simulink model "KD_cl_harness_tomasso"  (R2014b)
settings: Solver=ode45  StartTime=0  StopTime=50  FixedStep=0.01  MaxStep=0.005  RelTol=1e-4  AbsTol=1e-4
InitFcn:
  | load KD_const_coeffs_0624
  | load pexhat_stuff
  | load expcon
  | load thr_ff_map
values from neighbouring files (symbols this model uses):
  c_0 = 0    [expcon.mat]
  c_1 = 1    [expcon.mat]
  c_100 = 100    [expcon.mat]
  c_1000 = 1000    [expcon.mat]
  c_10000 = 10000    [expcon.mat]
  c_1000inv = 0.0010000000475    [expcon.mat]    (also in pexhat_stuff.mat)
  c_100inv = 0.00999999977648    [expcon.mat]
  c_1_int = 1    [expcon.mat]
  c_1d2p4 = 0.416666656733    [expcon.mat]
  c_1p7 = 1.70000004768    [expcon.mat]
  c_4400inv = 0.000227272728807    [pexhat_stuff.mat]
  c_5500inv = 0.000181818177225    [expcon.mat]
  c_80 = 80    [expcon.mat]
  c_90 = 90    [expcon.mat]
  c_cal_phi = 7.6395999713e-06    [expcon.mat]
  c_compmap = [28125.0058594 29577.4082031 31350.1035156 33776.21875 37051.9296875 41026.2695312 45453.9960938 50160.3515625 55029.671875 59986.109375 64980.4296875 69980.4375 ... (320 elements, 20x16)]    [expcon.mat]
  c_ctok = 273.149993896    [expcon.mat]
  c_fflow_max = inf    [expcon.mat]
  c_fflow_min = 0    [expcon.mat]
  c_filt = 0.949999988079    [expcon.mat]
  c_flowdiv = 9.99999974738e-05    [expcon.mat]
  c_flowmin = 0    [expcon.mat]
  c_flowmult = 10000    [expcon.mat]
  c_inf = inf    [expcon.mat]
  c_km1d2k = 0.142857149243    [expcon.mat]
  c_mm3tokgpers = 2.77333338516e-08    [expcon.mat]
  c_n1 = -1    [expcon.mat]
  c_p00001 = 9.99999974738e-06    [expcon.mat]
  c_p01 = 0.00999999977648    [pexhat_stuff.mat]
  c_p016 = 0.01600000076    [expcon.mat]
  c_p1429 = 0.142900004983    [expcon.mat]
  c_p1e9 = 9.99999971718e-10    [expcon.mat]
  c_p4167 = 0.416700005531    [expcon.mat]    (also in pexhat_stuff.mat = 0.416666656733)
  c_p4d1p4 = 0.285714298487    [expcon.mat]
  c_p5401 = 0.540099978447    [expcon.mat]
  c_p9 = 0.899999976158    [expcon.mat]
  c_pincomp = 97.4216003418    [expcon.mat]
  c_ra = 287.002807617    [expcon.mat]
  c_rair = 287.09979248    [expcon.mat]
  c_Rby1000 = 0.000287000002572    [expcon.mat]
  c_roacorr = 8.05689978733e-06    [expcon.mat]
  c_rpmtoradpers = 0.104719758034    [expcon.mat]
  c_svrthrottle1 = [0.924875080585 0.575991511345 0.0858279466629 0.820202827454 0.445821881294 0.509882986546 0.0428557097912 0.753634572029 0]    [expcon.mat]
  c_svrthrottle2 = [0.145454958081 0.14545533061 0.363636374474 0.509091556072 0.509090721607 0.509091317654 0.545454084873 0.618182241917 0.145454272628]    [expcon.mat]
  c_svrthrottlearg = 0.10000000149    [expcon.mat]
  c_svrthrottlebeta = [2282.12670898 -3239.46044922 -142.784469604 -2660.34570312 1434.34350586 4150.43994141 -1580.68164062 -1039.89575195 791.34588623]    [expcon.mat]
  c_ta_max = inf    [expcon.mat]
  c_ta_min = 270    [expcon.mat]
  c_V = 0.0077999997884    [expcon.mat]
  c_vnliftmax = 90    [expcon.mat]
  c_vnliftmin = 40    [expcon.mat]
  Coefs =     [KD_const_coeffs_0624.mat]    (also in pexhat_stuff.mat)
  const =     [KD_const_coeffs_0624.mat]    (also in pexhat_stuff.mat)
  const_exhat =     [pexhat_stuff.mat]
  eegr_map =     [expcon.mat]
  egrr_delay_init = 0    [expcon.mat]
  epim_map =     [expcon.mat]
  eplufin_ff_map =     [expcon.mat]
  expcon =     [expcon.mat]
  invta = [5 5 5 5 2.5 0 0 0 0 0 0 0 ... (240 elements, 16x15)]    [expcon.mat]
  invtacols = [1000 1200 1400 1600 1800 2000 2200 2400 2600 2800 3000 3200 ... (16 elements, 1x16)]    [expcon.mat]
  IV =     [KD_const_coeffs_0624.mat]    (also in pexhat_stuff.mat)
  Lobs_init = [0 0 0]    [expcon.mat]
  map_delay_init = 120    [expcon.mat]
  maxA_t = [51.4567184448 53.8593139648 56.3063011169 58.7576789856 61.1701469421 63.4982337952 65.6955718994 67.7161483765 69.5156555176 71.0527648926 72.2902603149 73.1961746216 ... (16 elements, 1x16)]    [expcon.mat]
  obsA = [0.985195398331  0  0; -0.188821405172  1  0; 0.000342977960827  0  1]    [expcon.mat]
  sample_time = 0.016    [expcon.mat]    (also in pexhat_stuff.mat)
  SVR_EGR =     [KD_const_coeffs_0624.mat]    (also in pexhat_stuff.mat)
  SVR_EGR_exhat =     [pexhat_stuff.mat]
  SVR_throttle =     [KD_const_coeffs_0624.mat]    (also in pexhat_stuff.mat)
  uz_init = [0 0]    [expcon.mat]
undefined symbols (not defined in the file or in its folder): k1_table, k2_table, maxL, minL, Newton, Raphson
libraries: simulink x5
(part 2 of 6)

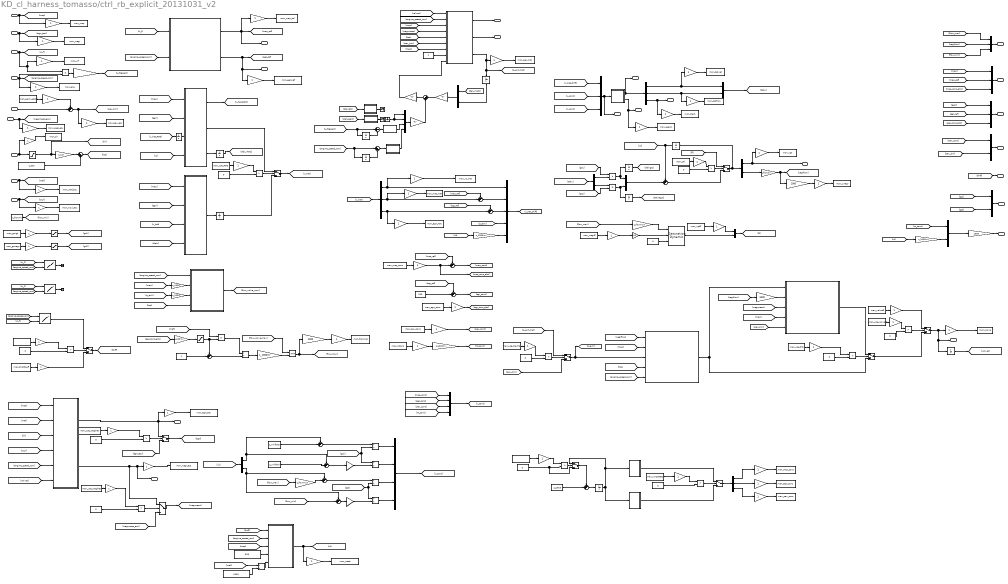
== system KD_cl_harness_tomasso/ctrl_rb_explicit_20131031_v2 ==
  map_kPa : Inport  OutDataTypeStr=single  PortDimensions=1  SampleTime=sample_time
  egrr_ecu : Inport  Port=2  OutDataTypeStr=single  PortDimensions=1  SampleTime=sample_time
  u_fuel_mm3pst : Inport  Port=3  OutDataTypeStr=single  PortDimensions=1  SampleTime=sample_time
  ene_rpm : Inport  Port=4  OutDataTypeStr=single  PortDimensions=1  SampleTime=sample_time
  pexh_kpa : Inport  Port=5  OutDataTypeStr=single  PortDimensions=1  SampleTime=sample_time
  t_in_C : Inport  Port=6  OutDataTypeStr=single  PortDimensions=1  SampleTime=sample_time
  wegrmeas_gps : Inport  Port=7  OutDataTypeStr=single  PortDimensions=1  SampleTime=sample_time
  maf_gps : Inport  Port=8  OutDataTypeStr=single  PortDimensions=1  SampleTime=sample_time
  wcyl : Inport  Port=9  OutDataTypeStr=single  PortDimensions=1  SampleTime=sample_time
  Data Store Read : DataStoreRead  DataStoreName=man_gsvgt  SampleTime=sample_time
  Data Store Read1 : DataStoreRead  DataStoreName=man_gswegr  SampleTime=sample_time
  Data Store Read10 : DataStoreRead  DataStoreName=man_use_valveff  SampleTime=sample_time
  Data Store Read11 : DataStoreRead  DataStoreName=man_valveff  SampleTime=sample_time
  Data Store Read12 : DataStoreRead  DataStoreName=man_use_throttleffmap  SampleTime=sample_time
  Data Store Read13 : DataStoreRead  DataStoreName=man_use_PexHat  SampleTime=sample_time
  Data Store Read14 : DataStoreRead  DataStoreName=man_pexh_adder  SampleTime=sample_time
  Data Store Read15 : DataStoreRead  DataStoreName=man_use_PID  SampleTime=sample_time
  Data Store Read16 : DataStoreRead  DataStoreName=man_use_ROO  SampleTime=sample_time
  Data Store Read17 : DataStoreRead  DataStoreName=man_pex_cons  SampleTime=sample_time
  Data Store Read18 : DataStoreRead  DataStoreName=man_ntcons  SampleTime=sample_time
  Data Store Read19 : DataStoreRead  DataStoreName=man_run2500tp  SampleTime=sample_time
  Data Store Read2 : DataStoreRead  DataStoreName=man_throttle_ff  SampleTime=sample_time
  Data Store Read20 : DataStoreRead  DataStoreName=man_start_pattern  SampleTime=sample_time
  Data Store Read3 : DataStoreRead  DataStoreName=man_map_cons  SampleTime=sample_time
  Data Store Read4 : DataStoreRead  DataStoreName=man_egrr_cons  SampleTime=sample_time
  Data Store Read5 : DataStoreRead  DataStoreName=man_vgtff  SampleTime=sample_time
  Data Store Read6 : DataStoreRead  DataStoreName=man_wegrff  SampleTime=sample_time
  Data Store Read7 : DataStoreRead  DataStoreName=man_ctrl  SampleTime=sample_time
  Data Store Read8 : DataStoreRead  DataStoreName=man_use_wegrhat  SampleTime=sample_time
  Data Store Read9 : DataStoreRead  DataStoreName=man_use_wegrhat  SampleTime=sample_time
  Data Store Write : DataStoreWrite  DataStoreName=mon_map
  Data Store Write1 : DataStoreWrite  DataStoreName=mon_wegr
  Data Store Write10 : DataStoreWrite  DataStoreName=mon_map_hat
  Data Store Write11 : DataStoreWrite  DataStoreName=mon_egrr_hat
  Data Store Write12 : DataStoreWrite  DataStoreName=mon_x1_hat
  Data Store Write13 : DataStoreWrite  DataStoreName=mon_flowmax
  Data Store Write14 : DataStoreWrite  DataStoreName=mon_delvgt
  Data Store Write15 : DataStoreWrite  DataStoreName=mon_delflow
  Data Store Write16 : DataStoreWrite  DataStoreName=mon_slack
  Data Store Write17 : DataStoreWrite  DataStoreName=mon_region
  Data Store Write18 : DataStoreWrite  DataStoreName=mon_vgt
  Data Store Write19 : DataStoreWrite  DataStoreName=mon_uwegr
  Data Store Write2 : DataStoreWrite  DataStoreName=mon_wf
  Data Store Write20 : DataStoreWrite  DataStoreName=mon_valve
  Data Store Write21 : DataStoreWrite  DataStoreName=mon_pex_hat
  Data Store Write22 : DataStoreWrite  DataStoreName=mon_wcyl_ecu
  Data Store Write23 : DataStoreWrite  DataStoreName=mon_egrr_est
  Data Store Write24 : DataStoreWrite  DataStoreName=mon_wegr_est
  Data Store Write25 : DataStoreWrite  DataStoreName=mon_ntest
  Data Store Write26 : DataStoreWrite  DataStoreName=man_map_cons
  Data Store Write27 : DataStoreWrite  DataStoreName=man_egrr_cons
  Data Store Write28 : DataStoreWrite  DataStoreName=man_pex_cons
  Data Store Write3 : DataStoreWrite  DataStoreName=mon_ene
  Data Store Write4 : DataStoreWrite  DataStoreName=mon_pex_ecu
  Data Store Write5 : DataStoreWrite  DataStoreName=mon_wegr_ecu
  Data Store Write6 : DataStoreWrite  DataStoreName=mon_tin
  Data Store Write7 : DataStoreWrite  DataStoreName=mon_maf_ecu
  Data Store Write8 : DataStoreWrite  DataStoreName=mon_map_ref
  Data Store Write9 : DataStoreWrite  DataStoreName=mon_egrr_ref
  Demux1 : Demux  Outputs=3
  Demux2 : Demux  Outputs=2
  Demux3 : Demux  Outputs=[size(obsA,1)-2 1 1]
  Demux4 : Demux  Outputs=2
  Demux5 : Demux  Outputs=2
  Demux6 : Demux  Outputs=3
  Divide{,2,4,6} (4 alike) : Product  Inputs=*/
  Divide1 : Product  Inputs=/*
  Divide3 : Product  Inputs=/*
  Divide5 : Product  Inputs=**
  EGR_max_flow : Subsystem
  Gain : Gain  Gain=c_flowdiv
      settings: AttributesFormatString=%<Gain>
  Gain1 : Gain  Gain=c_1000inv
      settings: AttributesFormatString=%<Gain>
  Gain10 : Gain  Gain=expcon.pexpred.b  Multiplication=Matrix(K*u) (u vector)
      settings: AttributesFormatString=%<Multiplication>
  Gain11 : Gain  Gain=expcon.pexpred.c  Multiplication=Matrix(K*u) (u vector)
      settings: AttributesFormatString=%<Multiplication>
  Gain12 : Gain  Gain=1000
      settings: AttributesFormatString=%<Gain>
  Gain2 : Gain  Gain=c_1000
      settings: AttributesFormatString=%<Gain>
  Gain3 : Gain  Gain=c_1000inv
      settings: AttributesFormatString=%<Gain>
  Gain4 : Gain  Gain=c_1000
      settings: AttributesFormatString=%<Gain>
  Gain5 : Gain  Gain=c_1000inv
      settings: AttributesFormatString=%<Gain>
  Gain6 : Gain  Gain=1000
      settings: AttributesFormatString=%<Gain>
  Gain7 : Gain  Gain=expcon.pexpred.a  Multiplication=Matrix(K*u) (u vector)
      settings: AttributesFormatString=%<Multiplication>
  Gain8 : Gain  Gain=c_1p7
      settings: AttributesFormatString=%<Gain>
  Gain9 : Gain  Gain=10
      settings: AttributesFormatString=%<Gain>
  Ground : Ground
  MinMax : MinMax  Inputs=2
      settings: AttributesFormatString=%<Function>
  Mux{,6,8..9} (4 alike) : Mux  Inputs=3
  Mux1 : Mux
  Mux{3,5,7,10..13} (7 alike) : Mux  Inputs=2
  Mux14 : Mux
  Mux2 : Mux  Inputs=5
  Mux4 : Mux
  PID : Subsystem  SystemSampleTime=.032
  Product : Product  RndMeth=Zero
  Product1 : Product  RndMeth=Zero
  Relational Operator{,1..9} (10 alike) : RelationalOperator  Operator=>  OutDataTypeStr=boolean
      settings: AttributesFormatString=%<Operator>
  Saturation1 : Saturate  UpperLimit=c_p9  LowerLimit=c_0
      settings: AttributesFormatString=%<LowerLimit>\n%<UpperLimit>
  Saturation2 : Saturate  UpperLimit=c_inf  LowerLimit=.125
      settings: AttributesFormatString=%<LowerLimit>\n%<UpperLimit>
  Saturation3 : Saturate  UpperLimit=c_inf  LowerLimit=.125
      settings: AttributesFormatString=%<LowerLimit>\n%<UpperLimit>
  Saturation5 : Saturate  UpperLimit=c_inf  LowerLimit=c_0
      settings: AttributesFormatString=%<LowerLimit>\n%<UpperLimit>
  Saturation_Dynamic1 : simulink/Discontinuities/Saturation Dynamic  OutMin=[]  OutMax=[]  OutDataTypeStr=Inherit: Same as second input  OutDataType=fixdt(1, 16)  OutScaling=2^-10  DoSatur=off
  Sum1 : Sum  Inputs=++|
  Sum10 : Sum  Inputs=++|
  Sum11 : Sum  Inputs=|++
  Sum12 : Sum  Inputs=|++
  Sum{2..9,13} (9 alike) : Sum  Inputs=-+|
  Sum14 : Sum  Inputs=|+-
  Sum15 : Sum  Inputs=|+-
  Sum16 : Sum  Inputs=++|
  Switch{,1..9} (10 alike) : Switch  Criteria=u2 ~= 0
      settings: AttributesFormatString=%<Criteria>
  Terminator : Terminator
  Terminator1 : Terminator
  Terminator_1 : Terminator
  Terminator_11 : Terminator
  Unit Delay : UnitDelay  InitialCondition=Lobs_init  SampleTime=-1
      settings: AttributesFormatString=%<X0>
  Unit Delay1 : UnitDelay  InitialCondition=uz_init  SampleTime=-1
      settings: AttributesFormatString=%<X0>
  Unit Delay{3..10} (8 alike) : UnitDelay  SampleTime=-1
      settings: AttributesFormatString=%<X0>
  Unit Delay2 : UnitDelay  InitialCondition=200  SampleTime=-1
      settings: AttributesFormatString=%<X0>
  While_Iterator_Subsystem : Subsystem  TreatAsAtomicUnit=on
  c_100inv : Gain  Gain=c_100inv
      settings: AttributesFormatString=%<Gain>
  ctok : Constant  Value=c_ctok  OutDataTypeStr=single  SampleTime=sample_time
      settings: AttributesFormatString=%<Value>\n%<SampleTime>
  custom_filter : Subsystem  Tag=FilterWizardSubSystem
      settings: ErrorFcn=dspFilterRealizedInBasicElemsAlgLoopErrFcnCallback
  custom_filter1 : Subsystem  Tag=FilterWizardSubSystem
      settings: ErrorFcn=dspFilterRealizedInBasicElemsAlgLoopErrFcnCallback
  custom_filter2 : Subsystem  Tag=FilterWizardSubSystem
      settings: ErrorFcn=dspFilterRealizedInBasicElemsAlgLoopErrFcnCallback
  custom_filter3 : Subsystem  Tag=FilterWizardSubSystem
      settings: ErrorFcn=dspFilterRealizedInBasicElemsAlgLoopErrFcnCallback
  egr_est : Subsystem
  expcon : Subsystem
  flowmin : Constant  Value=c_flowmin  OutDataTypeStr=single  SampleTime=sample_time
      settings: AttributesFormatString=%<Value>\n%<SampleTime>
  gain_schedule_egr : Lookup2D  RowIndex=thr_ff_fuel  ColumnIndex=thr_ff_ene  Table=k2_table  LookUpMeth=Interpolation-Use End Values
      settings: AttributesFormatString=%<LookUpMeth>\n%<RowIndex>\n%<ColumnIndex>
  gain_schedule_uvnlift : Lookup2D  RowIndex=thr_ff_fuel  ColumnIndex=thr_ff_ene  Table=k1_table  LookUpMeth=Interpolation-Use End Values
      settings: AttributesFormatString=%<LookUpMeth>\n%<RowIndex>\n%<ColumnIndex>
  invert_flow : Subsystem  SystemSampleTime=.032
  man_ctrl : Gain
  man_egrr_cons : Gain
  man_egrr_cons1 : Gain
  man_gsvgt : Gain
  man_gswegr : Gain
  man_map_cons : Gain
  man_map_cons1 : Gain
  man_ntcons : Gain
  man_pex_cons : Gain
  man_pex_cons1 : Gain
  man_pexh_adder : Gain
  man_run2500tp : Gain
  man_start_pattern : Gain
  man_throttle_ff : Gain
  man_use_PID : Gain
  man_use_PexHat : Gain
  man_use_ROO : Gain
  man_use_throttleffmap : Gain
  man_use_valveff : Gain
  man_use_wegrhat : Gain
  man_use_wegrhat2 : Gain
  man_valveff : Gain
  man_vgtff : Gain
  man_wegrff : Gain
  mon_delflow : Gain
  mon_delvgt : Gain
  mon_egrr_est : Gain
  mon_egrr_hat : Gain
  mon_egrr_ref : Gain
  mon_ene : Gain
  mon_flowmax : Gain
  mon_maf_ecu : Gain
  mon_map : Gain
  mon_map_hat : Gain
  mon_map_ref : Gain
  mon_ntest : Gain
  mon_pex_ecu : Gain
  mon_pex_hat : Gain
  mon_region : Gain  OutDataTypeStr=int32
  mon_slack : Gain
  mon_tin : Gain
  mon_uwegr : Gain
  mon_valve : Gain
  mon_vgt : Gain
  mon_wcyl_ecu : Gain
  mon_wegr : Gain
  mon_wegr_ecu : Gain
  mon_wegr_est : Gain
  mon_wf : Gain
  mon_x1_hat : Gain
  n1 : Gain  Gain=c_n1
      settings: AttributesFormatString=%<Gain>
  n2 : Gain  Gain=c_n1
      settings: AttributesFormatString=%<Gain>
  n3 : Gain  Gain=c_flowmult
      settings: AttributesFormatString=%<Gain>
  n4 : Gain  Gain=c_1000inv
      settings: AttributesFormatString=%<Gain>
  n5 : Gain  Gain=c_flowmult
      settings: AttributesFormatString=%<Gain>
  n6 : Gain  Gain=1000
      settings: AttributesFormatString=%<Gain>
  n7 : Gain  Gain=1000
      settings: AttributesFormatString=%<Gain>
  n9 : Gain  Gain=c_mm3tokgpers
      settings: AttributesFormatString=%<Gain>
  ntestimator : Subsystem  SystemSampleTime=.016
  obs : Subsystem
  product : Product  Inputs=**
  rate_max1 : Constant  OutDataTypeStr=single  SampleTime=sample_time
      settings: AttributesFormatString=%<Value>\n%<SampleTime>
  reduced_obs : Subsystem
  rpm1200testpattern : Subsystem
  rpm2500testpattern : Subsystem
  set_point_maps : Subsystem
  thousand : Constant  Value=1000  OutDataTypeStr=single  SampleTime=sample_time
      settings: AttributesFormatString=%<Value>\n%<SampleTime>
  thr_ff_map : Lookup2D  RowIndex=eplufin_ff_map.x  ColumnIndex=eplufin_ff_map.y  Table=eplufin_ff_map.z  LookUpMeth=Interpolation-Use End Values
      settings: AttributesFormatString=%<LookUpMeth>\n%<RowIndex>\n%<ColumnIndex>
  tic : Constant  Value=303  OutDataTypeStr=single  SampleTime=sample_time
      settings: AttributesFormatString=%<Value>\n%<SampleTime>
  vnliftmax : Constant  Value=c_vnliftmax  OutDataTypeStr=single  SampleTime=sample_time
      settings: AttributesFormatString=%<Value>\n%<SampleTime>
  vnliftmin : Constant  Value=c_vnliftmin  OutDataTypeStr=single  SampleTime=sample_time
      settings: AttributesFormatString=%<Value>\n%<SampleTime>
  y_cons1 : Constant  OutDataTypeStr=single  SampleTime=sample_time
      settings: AttributesFormatString=%<Value>\n%<SampleTime>
  y_cons5 : Constant  Value=100  OutDataTypeStr=single  SampleTime=sample_time
      settings: AttributesFormatString=%<Value>\n%<SampleTime>
  zero{,1..10} (11 alike) : Constant  Value=0  OutDataTypeStr=single  SampleTime=sample_time
      settings: AttributesFormatString=%<Value>\n%<SampleTime>
  zero11 : Constant  Value=c_p016  OutDataTypeStr=single  SampleTime=sample_time
      settings: AttributesFormatString=%<Value>\n%<SampleTime>
  u_vnlift : Outport  OutDataTypeStr=single
  u_egrflow : Outport  Port=2  OutDataTypeStr=single
  u_throttle : Outport  Port=3  OutDataTypeStr=single
  u_valve : Outport  Port=4  OutDataTypeStr=single
  slack : Outport  Port=5  OutDataTypeStr=single
  map_cons : Outport  Port=6  OutDataTypeStr=single
  egr_cons : Outport  Port=7  OutDataTypeStr=single
  region_num : Outport  Port=8  OutDataTypeStr=int32  PortDimensions=1
  map_ref : Outport  Port=9  OutDataTypeStr=single
  egr_ref : Outport  Port=10  OutDataTypeStr=single
  pex_cons : Outport  Port=11  OutDataTypeStr=single
  gs : Outport  Port=12  OutDataTypeStr=single
  nt_cons : Outport  Port=13  OutDataTypeStr=single
  expcon_in : Outport  Port=14  OutDataTypeStr=single
  expcon_out : Outport  Port=15  OutDataTypeStr=single
  pex_hat : Outport  Port=16  OutDataTypeStr=single
  dwdp : Outport  Port=17  OutDataTypeStr=single
  egr_rate_est : Outport  Port=18  OutDataTypeStr=single
  wegr : Outport  Port=19  OutDataTypeStr=single
  wires:
  mon_vgt/1 -> Data Store Write18/1
  [map] -> PID/4(p_in)
  [pex_sim] -> PID/5(p_ex)
  Switch6/1 -> Switch3/3
  PID/1(uvalve) -> Switch6/1
  zero7/1 -> Relational Operator6/2
  Data Store Read15/1 -> man_use_PID/1
  Relational Operator6/1 -> Switch6/2
  Sum10/1 -> [pex_sim], mon_pex_ecu/1
  pexh_kpa/1 -> Sum10/2
  Data Store Read14/1 -> man_pexh_adder/1
  Switch5/1 -> invert_flow/3(exhuast_pressure), [p_exh]
  zero6/1 -> Relational Operator5/2
  Data Store Read13/1 -> man_use_PexHat/1
  Relational Operator5/1 -> Switch5/2
  [wegrmeas] -> PID/3(wegr)
  Gain12/1 -> PID/2(uwegr)
  [uegrflow] -> Gain12/1
  Data Store Read2/1 -> man_throttle_ff/1
  zero5/1 -> Relational Operator4/2
  Data Store Read12/1 -> man_use_throttleffmap/1
  Relational Operator4/1 -> Switch4/2
  Data Store Read11/1 -> man_valveff/1
  Switch3/1 -> Unit Delay4/1, u_valve/1, mon_valve/1
  invert_flow/1(uvalve) -> Switch6/3, PID/1(valve_ff)
  zero4/1 -> Relational Operator3/2
  Data Store Read10/1 -> man_use_valveff/1
  Relational Operator3/1 -> Switch3/2
  n7/1 -> mon_uwegr/1
  n6/1 -> mon_flowmax/1
  Data Store Read8/1 -> man_use_wegrhat/1
  Relational Operator2/1 -> Switch1/2
  zero3/1 -> Relational Operator2/2
  Data Store Read9/1 -> man_use_wegrhat2/1
  Relational Operator1/1 -> Switch2/2
  zero2/1 -> Relational Operator1/2
  zero1/1 -> Relational Operator/2
  Data Store Read7/1 -> man_ctrl/1
  Relational Operator/1 -> Switch/2
  expcon/1(u_star) -> Demux1/1, expcon_out/1
  Mux/1 -> expcon/1(u), expcon_in/1
  [y_cons] -> Mux/3
  Demux1/3 -> slack/1, mon_slack/1
  Mux5/1 -> [delu]
  [u_cons] -> Mux/2
  [x_hat_shift] -> Mux/1
  [egrr] -> obs/2(egrr)
  [map] -> obs/1(map)
  [delu] -> obs/4(delu)
  obs/1(xhatp) -> Unit Delay/1
  [x_hat] -> obs/3(xhat)
  [flow_max] -> n3/1
  [flow_min] -> Sum5/2
  vnliftmax/1 -> Sum2/2
  Sum3/1 -> n1/1
  Demux4/2 -> Sum4/1, Sum5/1
  Sum5/1 -> n2/1
  n3/1 -> Sum4/2
  vnliftmin/1 -> Sum3/2
  Demux4/1 -> Sum2/1, Sum3/1
  [uz] -> Demux4/1
  Mux1/1 -> [u_cons]
  EGR_max_flow/1(mt_kg_per_sec) -> [flow_valve_max]
  [tico] -> EGR_max_flow/4(Tamb_K)
  [engine_speed_rpm] -> EGR_max_flow/1(Ne_rpm)
  [p_exh] -> Gain4/1
  [map] -> Gain2/1
  Gain4/1 -> EGR_max_flow/3(Pamb_Pa)
  Gain2/1 -> EGR_max_flow/2(Pim_Pa)
  [map_ref] -> Sum8/1
  [egr_ref] -> Sum9/1
  [x_hat] -> Demux3/1
  Mux2/1 -> [x_hat_shift]
  Sum9/1 -> Mux2/3
  Sum8/1 -> Mux2/2
  Demux3/3 -> Sum9/2, mon_egrr_hat/1
  Demux3/2 -> Sum8/2, mon_map_hat/1
  Demux3/1 -> Mux2/1, mon_x1_hat/1
  [uegrflow] -> Mux6/2
  [egrr] -> Mux9/1
  [map_ref] -> Mux8/2
  [map] -> Mux8/1
  Mux9/1 -> egr_cons/1
  Mux8/1 -> map_cons/1
  [flow_min] -> Mux6/3
  [flow_max] -> Mux6/1
  Mux6/1 -> u_egrflow/1
  [egr_ref] -> Mux9/2
  [uegrflow] -> invert_flow/1(valve_flow_command)
  [engine_speed_rpm] -> invert_flow/5(ne_rpm)
  [map] -> invert_flow/2(intake_pressure)
  [tico] -> invert_flow/4(Tintake)
  Unit Delay1/1 -> [uz], Sum1/1
  Gain/1 -> n7/1, [uegrflow]
  Demux2/2 -> Gain/1
  Demux2/1 -> mon_vgt/1, u_vnlift/1
  t_in_C/1 -> Saturation5/1, mon_tin/1
  ene_rpm/1 -> [engine_speed_rpm], Divide5/2, mon_ene/1
  flowmin/1 -> [flow_min]
  u_fuel_mm3pst/1 -> [w_f], Divide5/1, mon_wf/1
  egrr_ecu/1 -> [egrr_ecu], mon_wegr/1
  map_kPa/1 -> [map], mon_map/1
  expcon/2(region_num) -> region_num/1, mon_region/1
  set_point_maps/1(intake_pressure_ref) -> [map_ref], map_ref/1, mon_map_ref/1
  set_point_maps/2(EGR_ref) -> [egr_ref], egr_ref/1, mon_egrr_ref/1
  [w_f] -> set_point_maps/1(fuel_rate_mm3perst)
  [engine_speed_rpm] -> set_point_maps/2(engine_speed_rpm)
  Sum2/1 -> Divide/1
  Divide/1 -> Mux1/1
  [gs1] -> Divide/2, Divide1/1
  n1/1 -> Divide1/2
  Divide1/1 -> Mux1/2
  Divide2/1 -> Mux1/3
  [gs2] -> Divide2/2, Divide3/1
  n2/1 -> Divide3/2
  Divide3/1 -> Mux1/4
  [delu] -> Demux5/1
  Demux5/1 -> Product/2
  [gs1] -> Product/1
  Demux5/2 -> Product1/1
  [gs2] -> Product1/2
  Product/1 -> Mux3/1, Unit Delay6/1
  Product1/1 -> Mux3/2, Unit Delay7/1
  Mux3/1 -> Sum1/2
  [map_cons] -> Mux4/1
  Mux4/1 -> [y_cons]
  [map_cons_abs] -> Mux8/3
  [egr_cons] -> Mux4/2
  [egr_cons_abs] -> Mux9/3
  [p_exh] -> Mux2/4
  Data Store Read17/1 -> man_pex_cons/1
  Mux7/1 -> pex_cons/1
  [pex_cons] -> Mux4/3
  [pex_cons] -> Mux7/1
  [pex_sim] -> Mux7/2
  [gs1] -> Mux10/1
  [gs2] -> Mux10/2
  Mux10/1 -> gs/1
  [nt] -> Gain1/1
  Data Store Read18/1 -> man_ntcons/1
  Gain1/1 -> Mux2/5
  Gain3/1 -> [nt_cons]
  [nt_cons] -> Mux4/4
  [nt_cons] -> Mux11/1
  [nt] -> Gain5/1
  Mux11/1 -> Gain6/1
  Gain5/1 -> Mux11/2
  Demux1/2 -> Mux5/2, mon_delflow/1
  Demux1/1 -> Mux5/1, mon_delvgt/1
  [w_f] -> gain_schedule_uvnlift/1
  [engine_speed_rpm] -> gain_schedule_uvnlift/2
  [w_f] -> gain_schedule_egr/1
  [engine_speed_rpm] -> gain_schedule_egr/2
  gain_schedule_uvnlift/1 -> Terminator_11/1
  gain_schedule_egr/1 -> Terminator_1/1
  [engine_speed_rpm] -> thr_ff_map/1
  [w_f] -> thr_ff_map/2
  thr_ff_map/1 -> Switch4/1
  Sum4/1 -> Divide2/1
  wegrmeas_gps/1 -> [wegrmeas_ecu], mon_wegr_ecu/1
  ctok/1 -> Sum12/2
  Sum12/1 -> [tico]
  Gain8/1 -> Sum12/1
  [egr_ref] -> Sum7/1
  Data Store Read3/1 -> man_map_cons/1
  [map_ref] -> Sum6/1
  Sum6/1 -> [map_cons]
  Data Store Read4/1 -> man_egrr_cons/1
  Sum7/1 -> [egr_cons]
  maf_gps/1 -> [maf], mon_maf_ecu/1
  y_cons5/1 -> Sum7/2
  [maf] -> product/1
  product/1 -> Divide4/1
  rate_max1/1 -> Sum13/2
  Sum13/1 -> Divide4/2
  Divide4/1 -> n4/1
  [flow_valve_max] -> MinMax/1
  n4/1 -> MinMax/2
  MinMax/1 -> n6/1, [flow_max]
  Data Store Read1/1 -> man_gswegr/1
  Data Store Read/1 -> man_gsvgt/1
  [egr_cons_abs] -> c_100inv/1
  c_100inv/1 -> Saturation1/1
  Unit Delay4/1 -> [valvez]
  Saturation1/1 -> Sum13/1, product/2
  Data Store Read6/1 -> man_wegrff/1
  Data Store Read5/1 -> man_vgtff/1
  [flow_max] -> n5/1
  n5/1 -> Saturation_Dynamic1/1
  Gain9/1 -> Saturation_Dynamic1/2
  zero/1 -> Saturation_Dynamic1/3
  Saturation_Dynamic1/1 -> Mux13/2
  Mux13/1 -> [ff]
  [ff] -> Switch/1
  Sum1/1 -> Switch/3
  Switch/1 -> Unit Delay1/1, Demux2/1
  wcyl/1 -> [wcyl], mon_wcyl_ecu/1
  [maf] -> egr_est/2(maf)
  [tin] -> egr_est/3(tin)
  [wcyl] -> egr_est/4(wcyl)
  [engine_speed_rpm] -> egr_est/5(ene)
  egr_est/1(egrr) -> egr_rate_est/1, Switch1/1, mon_egrr_est/1
  [map] -> egr_est/1(pin)
  egr_est/2(wegr) -> Switch2/1, wegr/1, mon_wegr_est/1
  Switch1/1 -> [egrr]
  [egrr_ecu] -> Switch1/3
  Switch2/1 -> [wegrmeas]
  [wegrmeas_ecu] -> Switch2/3
  Saturation3/1 -> [gs1]
  Saturation2/1 -> [gs2]
  Saturation5/1 -> Gain8/1, [tin]
  [pex_sim] -> Switch5/3
  [p_exh_hat] -> Switch5/1
  [egrr] -> reduced_obs/2(egrr)
  [map] -> reduced_obs/1(map)
  [uz] -> reduced_obs/4(u)
  reduced_obs/1(xhatRO) -> [x_hat_ROO]
  [x_hat_ROO] -> Unit Delay5/1
  Unit Delay5/1 -> reduced_obs/3(xhatROpm1)
  zero8/1 -> Relational Operator7/2
  Data Store Read16/1 -> man_use_ROO/1
  Relational Operator7/1 -> Switch7/2
  Unit Delay/1 -> Switch7/3
  reduced_obs/2(xhat) -> Switch7/1
  Switch7/1 -> [x_hat]
  [valvez] -> egr_est/6(valve)
  [valvez] -> While_Iterator_Subsystem/1(In1)
  [engine_speed_rpm] -> While_Iterator_Subsystem/2(In2)
  [map] -> While_Iterator_Subsystem/3(In3)
  [wegrmeas] -> While_Iterator_Subsystem/4(In4)
  [tico] -> While_Iterator_Subsystem/5(In5)
  [pex_sim] -> While_Iterator_Subsystem/6(In6)
  [map] -> While_Iterator_Subsystem/7(In7)
  While_Iterator_Subsystem/1(Out1) -> pex_hat/1
  While_Iterator_Subsystem/2(Out2) -> dwdp/1
  While_Iterator_Subsystem/3(Out3) -> [p_exh_hat], Unit Delay2/1, mon_pex_hat/1
  y_cons1/1 -> While_Iterator_Subsystem/8(In8)
  Gain6/1 -> nt_cons/1
  Divide5/1 -> n9/1
  n9/1 -> [w_fkgpers]
  reduced_obs/3(delxhat) -> Unit Delay3/1
  [del_xhatz] -> Mux12/1
  Mux12/1 -> Gain7/1
  Gain7/1 -> Sum11/1
  Gain10/1 -> Sum11/2
  Mux14/1 -> Gain10/1
  Unit Delay6/1 -> [delvgtz]
  Unit Delay7/1 -> [delwegrz]
  Sum14/1 -> custom_filter/1(Input)
  [w_fkgpers] -> Sum14/1, Unit Delay8/1
  Unit Delay8/1 -> Sum14/2
  [engine_speed_rpm] -> Unit Delay9/1, Sum15/1
  Unit Delay9/1 -> Sum15/2
  Sum15/1 -> custom_filter1/1(Input)
  Sum11/1 -> Gain11/1
  custom_filter/1(Output) -> Mux14/3
  custom_filter1/1(Output) -> Mux14/4
  Gain11/1 -> While_Iterator_Subsystem/9(pexz)
  Unit Delay2/1 -> Mux12/2
  [delvgtz] -> custom_filter2/1(Input)
  [delwegrz] -> custom_filter3/1(Input)
  Ground/1 -> Mux14/2, Mux14/1
  custom_filter2/1(Output) -> Terminator/1
  custom_filter3/1(Output) -> Terminator1/1
  tic/1 -> ntestimator/4(T_out_IC)
  ntestimator/1(ntest) -> [nt], mon_ntest/1
  Switch4/1 -> [thrff]
  [thrff] -> u_throttle/1
  [engine_speed_rpm] -> ntestimator/2(omega_engine_rpm)
  [thrff] -> ntestimator/1(u_EGR_throttle)
  [map] -> ntestimator/3(p_intake_man)
  thousand/1 -> Divide6/2
  Divide6/1 -> ntestimator/5(maf)
  [maf] -> Divide6/1
  mon_map/1 -> Data Store Write/1
  mon_wegr/1 -> Data Store Write1/1
  mon_wf/1 -> Data Store Write2/1
  mon_ene/1 -> Data Store Write3/1
  man_pexh_adder/1 -> Sum10/1
  mon_pex_ecu/1 -> Data Store Write4/1
  mon_wegr_ecu/1 -> Data Store Write5/1
  mon_tin/1 -> Data Store Write6/1
  mon_maf_ecu/1 -> Data Store Write7/1
  mon_wcyl_ecu/1 -> Data Store Write22/1
  man_gsvgt/1 -> Saturation3/1
  man_gswegr/1 -> Saturation2/1
  man_use_throttleffmap/1 -> Relational Operator4/1
  man_throttle_ff/1 -> Switch4/3
  man_use_wegrhat/1 -> Relational Operator2/1
  mon_egrr_est/1 -> Data Store Write23/1
  mon_wegr_est/1 -> Data Store Write24/1
  man_use_wegrhat2/1 -> Relational Operator1/1
  mon_map_ref/1 -> Data Store Write8/1
  mon_egrr_ref/1 -> Data Store Write9/1
  Unit Delay3/1 -> [del_xhatz]
  man_use_ROO/1 -> Relational Operator7/1
  mon_flowmax/1 -> Data Store Write13/1
  mon_ntest/1 -> Data Store Write25/1
  man_ntcons/1 -> Gain3/1
  man_pex_cons/1 -> [pex_cons]
  man_egrr_cons/1 -> [egr_cons_abs]
  man_map_cons/1 -> Sum6/2, [map_cons_abs]
  mon_x1_hat/1 -> Data Store Write12/1
  mon_map_hat/1 -> Data Store Write10/1
  mon_egrr_hat/1 -> Data Store Write11/1
  mon_pex_hat/1 -> Data Store Write21/1
  mon_region/1 -> Data Store Write17/1
  mon_slack/1 -> Data Store Write16/1
  mon_delflow/1 -> Data Store Write15/1
  mon_delvgt/1 -> Data Store Write14/1
  man_ctrl/1 -> Relational Operator/1
  mon_uwegr/1 -> Data Store Write19/1
  man_wegrff/1 -> Gain9/1
  man_vgtff/1 -> Mux13/1
  man_use_PexHat/1 -> Relational Operator5/1
  man_use_PID/1 -> Relational Operator6/1
  man_valveff/1 -> Switch3/1
  man_use_valveff/1 -> Relational Operator3/1
  mon_valve/1 -> Data Store Write20/1
  Relational Operator8/1 -> Switch8/2
  zero9/1 -> Relational Operator8/2
  Data Store Read19/1 -> man_run2500tp/1
  rpm2500testpattern/1(Out4) -> Switch8/1
  rpm1200testpattern/1(Out4) -> Switch8/3
  Switch8/1 -> Demux6/1
  man_run2500tp/1 -> Relational Operator8/1
  man_map_cons1/1 -> Data Store Write26/1
  Demux6/1 -> man_map_cons1/1
  man_egrr_cons1/1 -> Data Store Write27/1
  Demux6/2 -> man_egrr_cons1/1
  man_pex_cons1/1 -> Data Store Write28/1
  Demux6/3 -> man_pex_cons1/1
  zero10/1 -> Relational Operator9/2, Switch9/3
  Data Store Read20/1 -> man_start_pattern/1
  man_start_pattern/1 -> Relational Operator9/1
  Relational Operator9/1 -> Switch9/2
  Sum16/1 -> Unit Delay10/1
  Unit Delay10/1 -> Switch9/1, rpm2500testpattern/1(In1), rpm1200testpattern/1(In1)
  Switch9/1 -> Sum16/1
  zero11/1 -> Sum16/2

== system KD_cl_harness_tomasso/pre-throttle manifold ==
  compressor_out : Inport
  intercooler_out : Inport  Port=2
  egr_throttle_out : Inport  Port=3
  Intake_man_out : Inport  Port=4
  Bus Creator : BusCreator  Inputs=1
  Bus Creator1 : BusCreator
  Bus Selector : BusSelector  OutputSignals=compressor_out.W_compressor,egr_throttle_out.W_EGR_Throttle,compressor_out.T_out_comp_sim,intercooler_out.T_out_IC
  p_preThrottle : Subsystem
  pre_throttle_out : Outport
  p_pre_throttle : Outport  Port=2
  wires:
  Bus Creator/1 -> pre_throttle_out/1  "pre_throttle_out"
  p_preThrottle/1("p_pre_throttle ") -> Bus Creator/1, p_pre_throttle/1  "p_pre_throttle"
  compressor_out/1 -> Bus Creator1/1
  intercooler_out/1 -> Bus Creator1/2
  egr_throttle_out/1 -> Bus Creator1/3
  Bus Creator1/1 -> Bus Selector/1
  Bus Selector/1 -> p_preThrottle/1(W_compressor)  "<W_compressor>"
  Bus Selector/2 -> p_preThrottle/2(W_throttle)  "<W_EGR_Throttle>"
  Bus Selector/3 -> p_preThrottle/3(T_out_compressor)  "<T_out_comp_sim>"
  Bus Selector/4 -> p_preThrottle/4(T_out_IC_data)  "<T_out_IC>"
  Intake_man_out/1 -> Bus Creator1/4

== system KD_cl_harness_tomasso/steps ==
  Constant : Constant
  Constant1 : Constant
  Constant2 : Constant  Value=2500
  From Workspace : FromWorkspace  VariableName=[0 5;10 55;20 5]  SampleTime=0  Interpolate=off  OutputAfterFinalValue=Holding final value
  Manual Switch : ManualSwitch
  Manual Switch1 : ManualSwitch  CurrentSetting=0
  Mux1 : Mux  Inputs=2
  Mux2 : Mux  Inputs=2
  Mux3 : Mux  Inputs=2
  Ne : simulink/Math Operations/Slider Gain  low=800  gain=2500  high=4000
  Subsystem : Subsystem  TreatAsAtomicUnit=on  SystemSampleTime=.032
  Subsystem1 : Subsystem  TreatAsAtomicUnit=on  SystemSampleTime=.032
  Subsystem2 : Subsystem  TreatAsAtomicUnit=on  SystemSampleTime=.032
  Uniform Random Number : UniformRandomNumber  Minimum=0  Maximum=60  SampleTime=5
  Uniform Random Number1 : UniformRandomNumber  Minimum=1000  Maximum=4000  SampleTime=50
  W_f : simulink/Math Operations/Slider Gain  low=0  gain=60  high=60
  Out1 : Outport
  wires:
  Constant/1 -> Ne/1
  Constant1/1 -> W_f/1
  W_f/1 -> Mux2/1
  Ne/1 -> Mux2/2
  Uniform Random Number1/1 -> Subsystem1/1(In1)
  Mux2/1 -> Manual Switch/1
  Mux1/1 -> Manual Switch/2
  Uniform Random Number/1 -> Subsystem/1(In1)
  Subsystem/1(Out1) -> Mux1/1
  Subsystem1/1(Out1) -> Mux1/2
  Manual Switch/1 -> Manual Switch1/1
  Manual Switch1/1 -> Out1/1
  Constant2/1 -> Mux3/2
  Subsystem2/1(Out1) -> Mux3/1
  From Workspace/1 -> Subsystem2/1(In1)
  Mux3/1 -> Manual Switch1/2

== system KD_cl_harness_tomasso/Combsution/Exhaust  ==
  omega_engine_radS : Inport
  T_intake_man : Inport  Port=2
  W_cyl : Inport  Port=3
  u_fuel : Inport  Port=4
  F1_in_man : Inport  Port=5
  Constant3 : Constant  Value=Coefs.ExhaustTemp
  MATLAB Function1 : MATLAB Function  TreatAsAtomicUnit=on
  conversion to RPM : Gain  Gain=30/pi
  T_exhaust : Outport
  wires:
  MATLAB Function1/1(T_exhaust) -> T_exhaust/1
  omega_engine_radS/1 -> conversion to RPM/1
  u_fuel/1 -> MATLAB Function1/4(u_fuel)
  F1_in_man/1 -> MATLAB Function1/5(F1_in)
  Constant3/1 -> MATLAB Function1/6(ExhaustTempCoefs)
  conversion to RPM/1 -> MATLAB Function1/1(omega_engine_rpm)
  T_intake_man/1 -> MATLAB Function1/2(T_in_man)
  W_cyl/1 -> MATLAB Function1/3(W_cyl)

== system KD_cl_harness_tomasso/Combsution/cylinder comp ==
  omega_engine_radS : Inport
  p_intake_man : Inport  Port=2
  p_exhaust_man : Inport  Port=3
  T_intake_man : Inport  Port=4
  T_exhaust_man : Inport  Port=5
  Constant : Constant  Value=const.Engine_Displacement_Volume_m3
  Constant1 : Constant  Value=const.R_specific_air_KJ_per_kg_kelvin
  Constant2 : Constant  Value=Coefs.CylFlow
  MATLAB Function : MATLAB Function  Priority=1  TreatAsAtomicUnit=on
  Mux : Mux  Inputs=2
  Terminator_3 : Terminator
  conversion to RPM : Gain  Gain=30/pi
  W_cyl_sim : Outport
  wires:
  Constant/1 -> Mux/1
  Mux/1 -> MATLAB Function/6(CylConstants)
  Constant1/1 -> Mux/2
  MATLAB Function/1(W_cyl_out) -> W_cyl_sim/1
  Constant2/1 -> MATLAB Function/7(cylFlowCoefs)
  omega_engine_radS/1 -> conversion to RPM/1
  conversion to RPM/1 -> MATLAB Function/1(omega_engine)
  p_intake_man/1 -> MATLAB Function/2(p_in_man)
  p_exhaust_man/1 -> MATLAB Function/3(p_exh_man)
  T_intake_man/1 -> MATLAB Function/4(T_in_man)
  T_exhaust_man/1 -> MATLAB Function/5(T_exh_man)
  MATLAB Function/2(nVol) -> Terminator_3/1

== system KD_cl_harness_tomasso/Compressor/Comp Map ==
  p_in_comp : Inport
  p_out_comp : Inport  Port=2
  T_in_comp_data : Inport  Port=3
  omega_turbo_data_radS : Inport  Port=4
  Constant : Constant  Value=const.compressor_diameter
  Constant1 : Constant  Value=const.Cp_Air_300K_J_per_kg_per_K
  Constant2 : Constant  Value=const.rho_Air_300K_kg_per_m3
  Constant3 : Constant  Value=const.gamma_air
  Constant4 : Constant  Value=const.R_specific_air_J_per_kg_kelvin
  Constant5 : Constant  Value=Coefs.CompPresRat
  Constant6 : Constant  Value=Coefs.CompEff
  Divide : Product  Inputs=/*
  MATLAB Function : MATLAB Function  TreatAsAtomicUnit=on
  Mux : Mux  Inputs=5
  Mux1 : Mux  Inputs=13
      settings: DisplayOption=signals
  Terminator_1 : Terminator
  Terminator_3 : Terminator
  conversion to RPM : Gain  Gain=30/pi
  W_comp_sim : Outport
  T_out_comp_sim : Outport  Port=2
  Tq_comp : Outport  Port=3
  wires:
  Mux/1 -> MATLAB Function/4(Comp_Constants)
  Constant5/1 -> MATLAB Function/5(CompPresRatCoefs)
  Constant6/1 -> MATLAB Function/6(CompEffCoefs)
  MATLAB Function/1(W_comp) -> W_comp_sim/1
  MATLAB Function/2(T_out_comp) -> T_out_comp_sim/1
  MATLAB Function/17(Tq_Compressor) -> Tq_comp/1
  MATLAB Function/4(pres_Rat1) -> Mux1/1
  MATLAB Function/5(Uc) -> Mux1/2
  MATLAB Function/6(Mach) -> Mux1/3
  MATLAB Function/7(psi) -> Mux1/4
  MATLAB Function/8(k1) -> Mux1/5
  MATLAB Function/9(k2) -> Mux1/6
  MATLAB Function/10(k3) -> Mux1/7
  MATLAB Function/11(PhiC) -> Mux1/8
  MATLAB Function/12(Comp_Efficiency) -> Mux1/9
  MATLAB Function/13(PhiC1) -> Mux1/10
  MATLAB Function/14(a1) -> Mux1/11
  MATLAB Function/15(a2) -> Mux1/12
  MATLAB Function/16(a3) -> Mux1/13
  p_in_comp/1 -> Divide/1
  p_out_comp/1 -> Divide/2
  Divide/1 -> MATLAB Function/1(pres_Rat)
  T_in_comp_data/1 -> MATLAB Function/2(T_in_comp)
  omega_turbo_data_radS/1 -> conversion to RPM/1
  conversion to RPM/1 -> MATLAB Function/3(omega_turbo_RPM)
  Constant/1 -> Mux/1
  Constant3/1 -> Mux/2
  Constant4/1 -> Mux/3
  Constant1/1 -> Mux/4
  Constant2/1 -> Mux/5
  Mux1/1 -> Terminator_1/1
  MATLAB Function/3(P_comp_W) -> Terminator_3/1

== system KD_cl_harness_tomasso/EGR Throttle/EGR Throttle ==
  u_EGR_throttle : Inport
  omega_engine_radS : Inport  Port=2
  p_intake_man : Inport  Port=3
  T_out_IC : Inport  Port=4
  p_preThrottle : Inport  Port=5
  Gain : Gain  Gain=1000
  Gain1 : Gain  Gain=1000
  Saturation : Saturate  UpperLimit=1  LowerLimit=0.001
  Terminator : Terminator
  Terminator1 : Terminator
  Throttle Model2 : Subsystem
  conversion to RPM : Gain  Gain=30/pi
  ThrottleFlow_kgpers : Outport
  wires:
  Throttle Model2/1(mt[kg/sec]) -> Saturation/1
  Throttle Model2/2(forwardmt[kg/sec]) -> Terminator/1
  u_EGR_throttle/1 -> Throttle Model2/1(TA[deg])
  omega_engine_radS/1 -> conversion to RPM/1
  p_intake_man/1 -> Gain/1
  T_out_IC/1 -> Throttle Model2/4(Tim[K]), Throttle Model2/6(Tamb[K])
  p_preThrottle/1 -> Gain1/1
  conversion to RPM/1 -> Throttle Model2/2(Ne[rpm])
  Gain/1 -> Throttle Model2/3(Pim[Pa])
  Gain1/1 -> Throttle Model2/5(Pamb[Pa])
  Throttle Model2/3(backwardmt[kg/sec]) -> Terminator1/1
  Saturation/1 -> ThrottleFlow_kgpers/1

== system KD_cl_harness_tomasso/EGR Valve/SVR EGR ==
  u_EGR_valve : Inport
  omega_engine_data_radS : Inport  Port=2
  p_intake_man_data : Inport  Port=3
  T_out_egr_cooler : Inport  Port=4
  p_exhaust_man_data : Inport  Port=5
  EGR_model : Subsystem
  Gain1 : Gain  Gain=1000
  Gain2 : Gain  Gain=1000
  Memory : Memory  X0=IV.T_out_egr_cooler  InheritSampleTime=on
  Terminator : Terminator
  conversion to RPM : Gain  Gain=30/pi
  EGR_kgpers : Outport
  wires:
  EGR_model/1(mt[kg/sec]) -> EGR_kgpers/1
  EGR_model/2(forwardmt[kg/sec]) -> Terminator/1
  u_EGR_valve/1 -> EGR_model/1(TA[deg])
  omega_engine_data_radS/1 -> conversion to RPM/1
  p_intake_man_data/1 -> Gain1/1
  T_out_egr_cooler/1 -> Memory/1
  p_exhaust_man_data/1 -> Gain2/1
  Gain1/1 -> EGR_model/3(Pim[Pa])
  Gain2/1 -> EGR_model/5(Pamb[Pa])
  conversion to RPM/1 -> EGR_model/2(Ne[rpm])
  Memory/1 -> EGR_model/4(Tim[K]), EGR_model/6(Tamb[K])

== system KD_cl_harness_tomasso/EGR cooler/EGR Cooler ==
  note: to reduce the numerical sensitivity
  T_exh_man : Inport
  T_coolant : Inport  Port=2
  W_egr_valve : Inport  Port=3
  u_EGR_cooler_bypass : Inport  Port=4
  omega_engine_data_radS : Inport  Port=5
  T_ambient : Inport  Port=6
  Constant : Constant  Value=Coefs.EGRCoolerTemp
  Constant1 : Constant  Value=Coefs.EGRCoolerbypassTemp
  Fcn3 : Fcn  Expr="Coefs.TinEGR(1)  + Coefs.TinEGR(2)*u(1) + Coefs.TinEGR(3)*u(2) + Coefs.TinEGR(4)*u(3) + Coefs.TinEGR(5)*u(1)^2 +Coefs.TinEGR(6)*u(2)^2"
  MATLAB Function : MATLAB Function  TreatAsAtomicUnit=on
  Mux3 : Mux  Inputs=3
  conversion to RPM1 : Gain  Gain=30/pi
  gain : Gain  Gain=1000
  T_out_EGR_cooler_sim : Outport
  W_egr_cooler : Outport  Port=2
  wires:
  Constant/1 -> MATLAB Function/6(EGRCoolerTempCoefs)
  Constant1/1 -> MATLAB Function/7(EGRCoolerbypassTempCoefs)
  MATLAB Function/1(T_out_EGR_cooler) -> T_out_EGR_cooler_sim/1
  T_coolant/1 -> MATLAB Function/2(T_coolant)
  u_EGR_cooler_bypass/1 -> MATLAB Function/4(EGRbypassflag)
  omega_engine_data_radS/1 -> conversion to RPM1/1
  conversion to RPM1/1 -> MATLAB Function/5(engine_speed_RPM)
  Fcn3/1 -> MATLAB Function/1(T_in_EGR_cooler)
  Mux3/1 -> Fcn3/1
  T_ambient/1 -> Mux3/3
  gain/1 -> Mux3/2
  W_egr_valve/1 -> W_egr_cooler/1, MATLAB Function/3(W_egr_valve), gain/1
  T_exh_man/1 -> Mux3/1

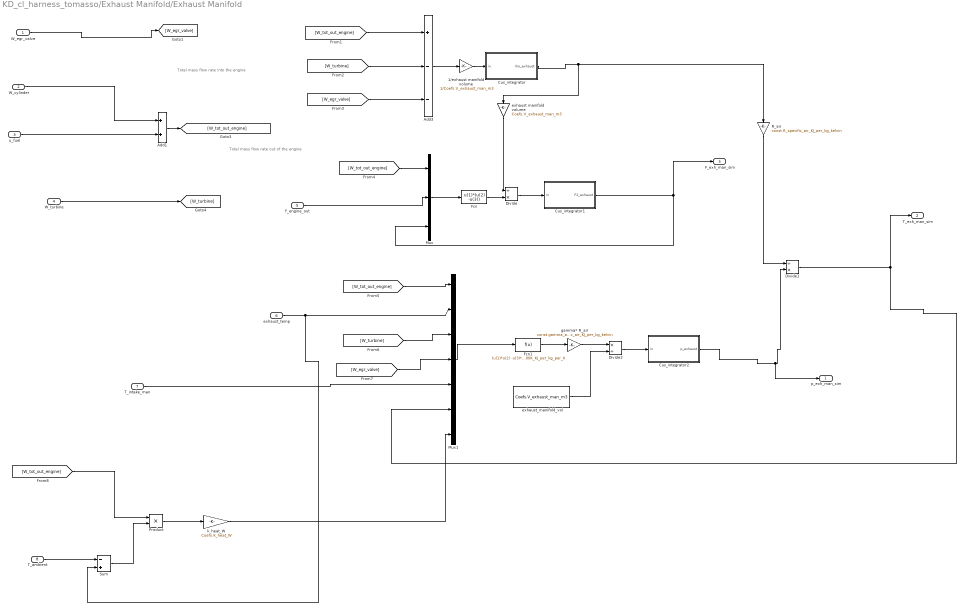
== system KD_cl_harness_tomasso/Exhaust Manifold/Exhaust Manifold ==
  note: Total mass flow rate into the engine
  note: Total mass flow rate out of the engine
  W_egr_valve : Inport
  W_cylinder : Inport  Port=2
  u_fuel : Inport  Port=3
  W_turbine : Inport  Port=4
  F_engine_out : Inport  Port=5
  exhaust_temp : Inport  Port=6
  T_intake_man : Inport  Port=7
  T_ambient : Inport  Port=8
  " R_air" : Gain  Gain=const.R_specific_air_KJ_per_kg_kelvin
  1/exhaust manifold volume : Gain  Gain=1/Coefs.V_exhaust_man_m3
  Add1 : Sum
  Add3 : Sum  Inputs=+--
  Cus_integrator : Subsystem
  Cus_integrator1 : Subsystem
  Cus_integrator2 : Subsystem
  Divide : Product  Inputs=/*
  Divide1 : Product  Inputs=/*
  Divide2 : Product  Inputs=*/
  Fcn : Fcn  Expr=u(1)*(u(2) -u(3))
  Fcn1 : Fcn  Expr=(u(1)*u(2) -u(3)*u(6) -u(4)*u(6)) - u(7)/const.Cp_Air_300K_KJ_per_kg_per_K
  Mux : Mux  Inputs=3
  Mux1 : Mux  Inputs=7
  Product : Product  RndMeth=Zero
  Sum : Sum  Inputs=-+
  exhaust manifold volume : Gain  Gain=Coefs.V_exhaust_man_m3
  exhaust_manifold_vol : Constant  Value=Coefs.V_exhaust_man_m3
  gamma* R_air : Gain  Gain=const.gamma_air*const.R_specific_air_KJ_per_kg_kelvin
  k_heat_W : Gain  Gain=Coefs.K_heat_W
  p_exh_man_sim : Outport
  T_exh_man_sim : Outport  Port=2
  F_exh_man_sim : Outport  Port=3
  wires:
  Add1/1 -> [W_tot_out_engine]
  [W_tot_out_engine] -> Add3/1
  [W_turbine] -> Add3/2
  [W_egr_valve] -> Add3/3
  Add3/1 -> 1/exhaust manifold volume/1
  1/exhaust manifold volume/1 -> Cus_integrator/1(in)
  [W_tot_out_engine] -> Mux/1
  F_engine_out/1 -> Mux/2
  Mux/1 -> Fcn/1
  Fcn/1 -> Divide/2
  exhaust manifold volume/1 -> Divide/1
  Divide/1 -> Cus_integrator1/1(in)
  Cus_integrator1/1(F2_exhaust) -> Mux/3, F_exh_man_sim/1
  Mux1/1 -> Fcn1/1
  gamma* R_air/1 -> Divide2/1
  Fcn1/1 -> gamma* R_air/1
  Cus_integrator2/1(p_exhaust) -> p_exh_man_sim/1, Divide1/2
  " R_air"/1 -> Divide1/1
  Divide1/1 -> Mux1/6, T_exh_man_sim/1
  Divide2/1 -> Cus_integrator2/1(in)
  exhaust_manifold_vol/1 -> Divide2/2
  Cus_integrator/1(rho_exhaust) -> exhaust manifold volume/1, " R_air"/1
  [W_tot_out_engine] -> Mux1/1
  [W_turbine] -> Mux1/3
  [W_egr_valve] -> Mux1/4
  exhaust_temp/1 -> Mux1/2, Sum/2
  W_cylinder/1 -> Add1/1
  W_egr_valve/1 -> [W_egr_valve]
  u_fuel/1 -> Add1/2
  W_turbine/1 -> [W_turbine]
  T_intake_man/1 -> Mux1/5
  Product/1 -> k_heat_W/1
  T_ambient/1 -> Sum/1
  [W_tot_out_engine] -> Product/1
  Sum/1 -> Product/2
  k_heat_W/1 -> Mux1/7

== system KD_cl_harness_tomasso/Intake Manifold/Intake_manifold ==
  note: Total mass flow rate into the engine
  W_throttle : Inport
  W_egr_valve : Inport  Port=2
  W_cyl_in : Inport  Port=3
  F2_exhaust_sim : Inport  Port=4
  T_out_egr_cooler : Inport  Port=5
  T_out_IC : Inport  Port=6
  " R_air1" : Gain  Gain=const.R_specific_air_KJ_per_kg_kelvin
  1/intake manifold volume : Gain  Gain=1/Coefs.V_intake_man_m3
  Add1 : Sum  Inputs=++-
  Cus_integrator : Subsystem
  Cus_integrator1 : Subsystem
  Cus_integrator2 : Subsystem
  Divide : Product  Inputs=/*
  Divide1 : Product  Inputs=/*
  Divide2 : Product  Inputs=*/
  Fcn : Fcn  Expr=u(3)*(u(2) - u(1)) - u(4)*u(1)
  Fcn1 : Fcn  Expr=u(1)*u(4) +u(2)*u(5) - u(6)*u(3)
  Intake_manifold_vol : Constant  Value=Coefs.V_intake_man_m3
  Mux : Mux
  Mux1 : Mux  Inputs=6
  gamma* R_air : Gain  Gain=const.gamma_air*const.R_specific_air_KJ_per_kg_kelvin
  intake manifold volume 1 : Gain  Gain=Coefs.V_intake_man_m3
  p_in_man_sim : Outport
  T_in_man_sim : Outport  Port=2
  F_in_man_sim : Outport  Port=3
  wires:
  Add1/1 -> 1/intake manifold volume/1
  1/intake manifold volume/1 -> Cus_integrator/1(in)
  [W_throttle] -> Add1/1
  [W_egr_valve] -> Add1/2
  [W_tot_in_engine] -> Add1/3
  Cus_integrator1/1(F1_intake) -> Mux/1, F_in_man_sim/1
  [W_egr_valve] -> Mux/3
  [W_throttle] -> Mux/4
  Mux/1 -> Fcn/1
  intake manifold volume 1/1 -> Divide/1
  Divide/1 -> Cus_integrator1/1(in)
  [W_throttle] -> Mux1/1
  [W_egr_valve] -> Mux1/2
  [W_tot_in_engine] -> Mux1/3
  Fcn/1 -> Divide/2
  Mux1/1 -> Fcn1/1
  Fcn1/1 -> gamma* R_air/1
  gamma* R_air/1 -> Divide2/1
  Divide2/1 -> Cus_integrator2/1(in)
  Divide1/1 -> T_in_man_sim/1, Mux1/6
  Intake_manifold_vol/1 -> Divide2/2
  " R_air1"/1 -> Divide1/1
  Cus_integrator/1(rho_intake) -> intake manifold volume 1/1, " R_air1"/1  "rho_intake"
  Cus_integrator2/1(p_intake) -> Divide1/2, p_in_man_sim/1
  F2_exhaust_sim/1 -> Mux/2
  T_out_IC/1 -> Mux1/4
  T_out_egr_cooler/1 -> Mux1/5
  W_throttle/1 -> [W_throttle]
  W_egr_valve/1 -> [W_egr_valve]
  W_cyl_in/1 -> [W_tot_in_engine]

== system KD_cl_harness_tomasso/Intercooler/Intercooler ==
  T_out_comp : Inport
  p_out_comp : Inport  Port=2
  T_ambient : Inport  Port=3
  Constant : Constant  Value=Coefs.ICTemp
  MATLAB Function : MATLAB Function  TreatAsAtomicUnit=on
  T_out_IC : Outport
  p_out_IC : Outport  Port=2
  wires:
  Constant/1 -> MATLAB Function/3(ICTempCoefs)
  T_out_comp/1 -> MATLAB Function/1(T_in_IC)
  MATLAB Function/1(T_out_IC) -> T_out_IC/1
  p_out_comp/1 -> p_out_IC/1
  T_ambient/1 -> MATLAB Function/2(T_ambient)

== system KD_cl_harness_tomasso/Turbine/TurbineMap ==
  note: from TC_0605
  omega_turbo_radS : Inport
  p_exhaust_man : Inport  Port=2
  T_ambient : Inport  Port=3
  T_exhaust_man : Inport  Port=4
  u_VGT : Inport  Port=5
  Constant11 : Constant  Value=const.gamma_air
  Constant12 : Constant  Value=const.Engine_Displacement_Volume_m3
  Constant13 : Constant  Value=const.Cp_Air_300K_J_per_kg_per_K
  Constant7 : Constant  Value=const.turbine_diameter
  Constant8 : Constant  Value=Coefs.TurbFlow
  Constant9 : Constant  Value=Coefs.TurbTemp
  Divide : Product  Inputs=*/
  Fcn3 : Fcn  Expr=Coefs.postTurbine(1)*u(1)^2 + Coefs.postTurbine(2)*u(1) + Coefs.postTurbine(3)
  Memory : Memory  X0=IV.W_turbine  InheritSampleTime=on
  Mux3 : Mux
  Terminator_{1..4} (4 alike) : Terminator
  TurbineMAP1 : MATLAB Function  Priority=2  TreatAsAtomicUnit=on
  conversion to RPM : Gain  Gain=30/pi
  W_out_turb_sim : Outport
  T_out_turb_sim : Outport  Port=2
  Tq_turbine : Outport  Port=3
  wires:
  omega_turbo_radS/1 -> conversion to RPM/1
  conversion to RPM/1 -> TurbineMAP1/2(omega_turbo)
  Constant12/1 -> Mux3/4
  Constant11/1 -> Mux3/3
  Constant7/1 -> Mux3/1
  Mux3/1 -> TurbineMAP1/7(Turb_Constants)
  Constant8/1 -> TurbineMAP1/8(TurbFlowCoefs)
  Constant9/1 -> TurbineMAP1/9(TurbTempCoefs)
  TurbineMAP1/1(W_turbine_sim) -> Memory/1, W_out_turb_sim/1
  TurbineMAP1/2(T_out_turbine) -> T_out_turb_sim/1
  TurbineMAP1/7(Tq_turbine) -> Tq_turbine/1
  Divide/1 -> TurbineMAP1/1(turb_pres_ratio)
  Fcn3/1 -> Divide/1
  p_exhaust_man/1 -> TurbineMAP1/3(p_in_turb), Divide/2
  Constant13/1 -> Mux3/2
  Memory/1 -> Fcn3/1
  T_ambient/1 -> TurbineMAP1/4(T_ambient)
  u_VGT/1 -> TurbineMAP1/6(VNlift)
  T_exhaust_man/1 -> TurbineMAP1/5(T_exh_man)
  TurbineMAP1/3(eta_turb) -> Terminator_3/1
  TurbineMAP1/4(A_turbine) -> Terminator_1/1
  TurbineMAP1/5(phi) -> Terminator_2/1
  TurbineMAP1/6(delta_T_Turbo) -> Terminator_4/1

== system KD_cl_harness_tomasso/Turbo Rotational Dynamics/Turbo rot ==
  note: stop simulation if turbo speed reaches below 1000 rad/sec
  Tq_compressor : Inport
  Tq_turbine : Inport  Port=2
  1/J_turbo : Gain  Gain=1/Coefs.J_turbo
  Compare To Constant : simulink/Logic and Bit Operations/Compare To Constant  relop=<=  const=1000  OutDataTypeStr=boolean
  Cus_integrator : Subsystem
  Stop Simulation : Stop
  Subtract : Sum  Inputs=--+
  To Workspace15 : ToWorkspace  VariableName=Tq_friction  SampleTime=-1
  Tq_friction : Fcn  Expr=Coefs.Tq_fNT(1) * u(1)^2 + Coefs.Tq_fNT(2) * u(1) + Coefs.Tq_fNT(3)
  Omega_turbo_radS : Outport
  wires:
  Subtract/1 -> 1/J_turbo/1
  1/J_turbo/1 -> Cus_integrator/1(delta_torque)
  Cus_integrator/1(NT_radS) -> Tq_friction/1, Compare To Constant/1, Omega_turbo_radS/1  "omega_turbo_radS"
  Tq_compressor/1 -> Subtract/2
  Tq_turbine/1 -> Subtract/3
  Tq_friction/1 -> To Workspace15/1, Subtract/1
  Compare To Constant/1 -> Stop Simulation/1

== system KD_cl_harness_tomasso/ctrl_rb_explicit_20131031_v2/EGR_max_flow ==
  Ne_rpm : Inport
  Pim_Pa : Inport  Port=2
  Pamb_Pa : Inport  Port=3
  Tamb_K : Inport  Port=4
  Air_Model_map_use : Subsystem
  Ra : Constant  Value=c_ra  OutDataTypeStr=single
      settings: AttributesFormatString=%<Value>
  mt_kg_per_sec : Outport
  wires:
  Ne_rpm/1 -> Air_Model_map_use/1(Ne_rpm)
  Ra/1 -> Air_Model_map_use/5(R_a)
  Air_Model_map_use/1(mt_kg_per_sec) -> mt_kg_per_sec/1
  Pim_Pa/1 -> Air_Model_map_use/2(Pim_Pa)
  Tamb_K/1 -> Air_Model_map_use/4(Ta_K)
  Pamb_Pa/1 -> Air_Model_map_use/3(Pa_Pa)
